simulink model "DFADAS2_SenFus_v1_201204RC_training_210115"  (R2018b)
settings: Solver=FixedStepDiscrete  StartTime=0.0  StopTime=inf  FixedStep=0.002  RelTol=1e-3  EnableMultiTasking=on
PreLoadFcn:
  | RTWConfigurationCB('preloadfcn', bdroot);
libraries: canmsglib x108, simulink x48, canfdmsglib x12
(part 20 of 28)

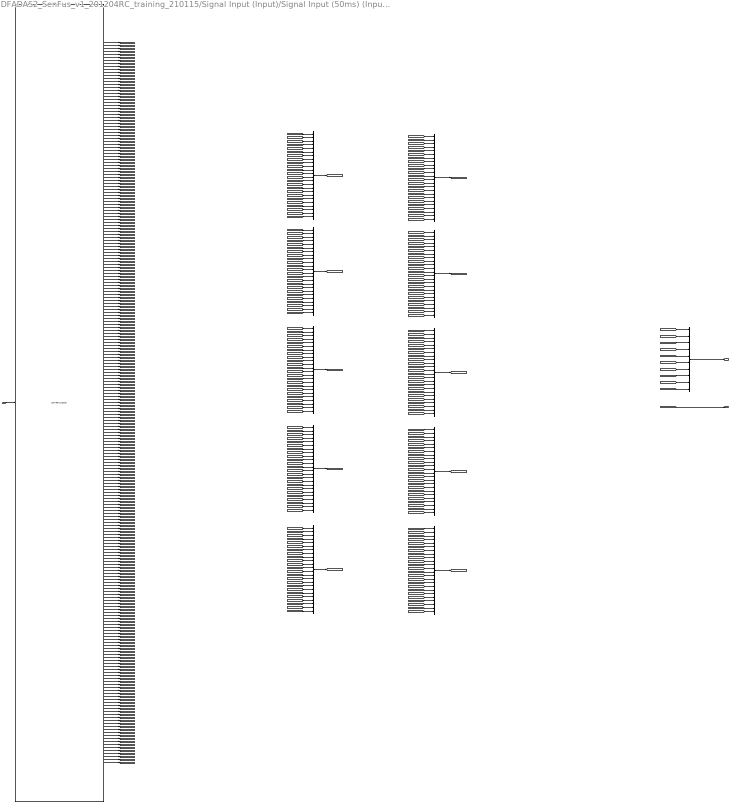
== system DFADAS2_SenFus_v1_201204RC_training_210115/Signal Input (Input)/Signal Input (50ms) (Input50)/Front Left Radar(S2) Objects Information (FLRdr)/S0 Data Frame Read/Enabled Subsystem/Unpack/If Action Subsystem/Unpack ==
  msg : Inport
  Bus Creator : BusCreator  Inputs=10
  Bus Creator{1..10} (10 alike) : BusCreator  Inputs=24
  CAN FD Unpack3 : canfdmsglib/CAN FD Unpack  CANdbFile=C:\Users\ThinkPad\Desktop\200529-海拉角雷达DBC\PR53671_DFPV_D53_HWA_SDE_F-SRR_CANFD_DF RESEARCH.dbc  MsgList=Object_Data_S2  MsgName=Object_Data_S2  ProtocolMode=CAN FD  MsgIDType=Standard (11-bit identifier)  MsgIdentifier=855  MsgLength=64  SignalInfo=ClassHighestProb_S2_001$135$7$1$2$3$0$1.000000e-02$0$-Inf$Inf$#ClassHighestProb_S2_002$323$7$1$2$3$0$1.000000e-02$0$-Inf$Inf$#ClassHighestProb_S2_003$135$7$1$2$3$1$1.000000e-02$0$-Inf$Inf$#ClassHighestProb_S2_004$323$7$1$2$3$1$1.000000e-02$0$-Inf$Inf$#ClassHighestProb_S2_005$135$7$1$2$3$2$1.000000e-02$0$-Inf$Inf$#ClassHighestProb_S2_006$323$7$1$2$3$2$1.000000e-02$0$-Inf$Inf$#ClassHighestProb_S2_007$135$7$1$2$3$3$1.000000e-02$0$-Inf$Inf$#ClassHighestProb_S2_008$323$7$1$2$3$3$1.000000e-02$0$-Inf$Inf$#ClassHighestProb_S2_009$135$7$1$2$3$4$1.000000e-02$0$-Inf$Inf$#ClassHighestProb_S2_010$323$7$1$2$3$4$1.000000e-02$0$-Inf$Inf$#ClassHighest_S2_001$132$3$1$2$3$0$1$0$0$7$#ClassHighest_S2_002$320$3$1$2$3$0$1$0$0$7$#ClassHighest_S2_003$132$3$1$2$3$1$1$0$0$7$#ClassHighest_S2_004$320$3$1$2$3$1$1$0$0$7$#ClassHighest_S2_005$132$3$1$2$3$2$1$0$0$7$#ClassHighest_S2_006$320$3$1$2$3$2$1$0$0$7$#ClassHighest_S2_007$132$3$1$2$3$3$1$0$0$7$#ClassHighest_S2_008$320$3$1$2$3$3$1$0$0$7$#ClassHighest_S2_009$132$3$1$2$3$4$1$0$0$7$#ClassHighest_S2_010$320$3$1$2$3$4$1$0$0$7$#ExistenceProbability_S2_001$121$7$1$2$3$0$1.000000e-02$0$0$1$#ExistenceProbability_S2_002$309$7$1$2$3$0$1.000000e-02$0$0$1$#ExistenceProbability_S2_003$121$7$1$2$3$1$1.000000e-02$0$0$1$#ExistenceProbability_S2_004$309$7$1$2$3$1$1.000000e-02$0$0$1$#ExistenceProbability_S2_005$121$7$1$2$3$2$1.000000e-02$0$0$1$#ExistenceProbability_S2_006$309$7$1$2$3$2$1.000000e-02$0$0$1$#ExistenceProbability_S2_007$121$7$1$2$3$3$1.000000e-02$0$0$1$#ExistenceProbability_S2_008$309$7$1$2$3$3$1.000000e-02$0$0$1$#ExistenceProbability_S2_009$121$7$1$2$3$4$1.000000e-02$0$0$1$#ExistenceProbability_S2_010$309$7$1$2$3$4$1.000000e-02$0$0$1$#Height_S2_001$146$6$1$2$3$0$1.000000e-01$0$0$5$#Height_S2_002$334$6$1$2$3$0$1.000000e-01$0$0$5$#Height_S2_003$146$6$1$2$3$1$1.000000e-01$0$0$5$#Height_S2_004$334$6$1$2$3$1$1.000000e-01$0$0$5$#Height_S2_005$146$6$1$2$3$2$1.000000e-01$0$0$5$#Height_S2_006$334$6$1$2$3$2$1.000000e-01$0$0$5$#Height_S2_007$146$6$1$2$3$3$1.000000e-01$0$0$5$#Height_S2_008$334$6$1$2$3$3$1.000000e-01$0$0$5$#Height_S2_009$146$6$1$2$3$4$1.000000e-01$0$0$5$#Height_S2_010$334$6$1$2$3$4$1.000000e-01$0$0$5$#Id_S2_001$8$10$1$2$3$0$1$1$1$1023$#Id_S2_002$196$10$1$2$3$0$1$1$1$1023$#Id_S2_003$8$10$1$2$3$1$1$1$1$1023$#Id_S2_004$196$10$1$2$3$1$1$1$1$1023$#Id_S2_005$8$10$1$2$3$2$1$1$1$1023$#Id_S2_006$196$10$1$2$3$2$1$1$1$1023$#Id_S2_007$8$10$1$2$3$3$1$1$1$1023$#Id_S2_008$196$10$1$2$3$3$1$1$1$1023$#Id_S2_009$8$10$1$2$3$4$1$1$1$1023$#Id_S2_010$196$10$1$2$3$4$1$1$1$1023$#Length_S2_001$102$9$1$2$3$0$1.000000e-01$0$3.000000e-01$5.140000e+01$#Length_S2_002$290$9$1$2$3$0$1.000000e-01$0$3.000000e-01$5.140000e+01$#Length_S2_003$102$9$1$2$3$1$1.000000e-01$0$3.000000e-01$5.140000e+01$#Length_S2_004$290$9$1$2$3$1$1.000000e-01$0$3.000000e-01$5.140000e+01$#Length_S2_005$102$9$1$2$3$2$1.000000e-01$0$3.000000e-01$5.140000e+01$#Length_S2_006$290$9$1$2$3$2$1.000000e-01$0$3.000000e-01$5.140000e+01$#Length_S2_007$102$9$1$2$3$3$1.000000e-01$0$3.000000e-01$5.140000e+01$#Length_S2_008$290$9$1$2$3$3$1.000000e-01$0$3.000000e-01$5.140000e+01$#Length_S2_009$102$9$1$2$3$4$1.000000e-01$0$3.000000e-01$5.140000e+01$#Length_S2_010$290$9$1$2$3$4$1.000000e-01$0$3.000000e-01$5.140000e+01$#MovingState_S2_001$128$4$1$2$3$0$1$0$0$15$#MovingState_S2_002$316$4$1$2$3$0$1$0$0$15$#MovingState_S2_003$128$4$1$2$3$1$1$0$0$15$#MovingState_S2_004$316$4$1$2$3$1$1$0$0$15$#MovingState_S2_005$128$4$1$2$3$2$1$0$0$15$#MovingState_S2_006$316$4$1$2$3$2$1$0$0$15$#MovingState_S2_007$128$4$1$2$3$3$1$0$0$15$#MovingState_S2_008$316$4$1$2$3$3$1$0$0$15$#MovingState_S2_009$128$4$1$2$3$4$1$0$0$15$#MovingState_S2_010$316$4$1$2$3$4$1$0$0$15$#Multiplexor$0$8$1$2$2$0$1$0$0$255$#ObjInit_S2_001$18$1$1$2$3$0$1$0$0$1$#ObjInit_S2_002$206$1$1$2$3$0$1$0$0$1$#ObjInit_S2_003$18$1$1$2$3$1$1$0$0$1$#ObjInit_S2_004$206$1$1$2$3$1$1$0$0$1$#ObjInit_S2_005$18$1$1$2$3$2$1$0$0$1$#ObjInit_S2_006$206$1$1$2$3$2$1$0$0$1$#ObjInit_S2_007$18$1$1$2$3$3$1$0$0$1$#ObjInit_S2_008$206$1$1$2$3$3$1$0$0$1$#ObjInit_S2_009$18$1$1$2$3$4$1$0$0$1$#ObjInit_S2_010$206$1$1$2$3$4$1$0$0$1$#ObjMeasured_S2_001$19$1$1$2$3$0$1$0$0$1$#ObjMeasured_S2_002$207$1$1$2$3$0$1$0$0$1$#ObjMeasured_S2_003$19$1$1$2$3$1$1$0$0$1$#ObjMeasured_S2_004$207$1$1$2$3$1$1$0$0$1$#ObjMeasured_S2_005$19$1$1$2$3$2$1$0$0$1$#ObjMeasured_S2_006$207$1$1$2$3$2$1$0$0$1$#ObjMeasured_S2_007$19$1$1$2$3$3$1$0$0$1$#ObjMeasured_S2_008$207$1$1$2$3$3$1$0$0$1$#ObjMeasured_S2_009$19$1$1$2$3$4$1$0$0$1$#ObjMeasured_S2_010$207$1$1$2$3$4$1$0$0$1$#Orientation_S2_001$111$10$1$2$3$0$1.000000e-02$-3.140000e+00$-3.140000e+00$3.140000e+00$#Orientation_S2_002$299$10$1$2$3$0$1.000000e-02$-3.140000e+00$-3.140000e+00$3.140000e+00$#Orientation_S2_003$111$10$1$2$3$1$1.000000e-02$-3.140000e+00$-3.140000e+00$3.140000e+00$#Orientation_S2_004$299$10$1$2$3$1$1.000000e-02$-3.140000e+00$-3.140000e+00$3.140000e+00$#Orientation_S2_005$111$10$1$2$3$2$1.000000e-02$-3.140000e+00$-3.140000e+00$3.140000e+00$#Orientation_S2_006$299$10$1$2$3$2$1.000000e-02$-3.140000e+00$-3.140000e+00$3.140000e+00$#Orientation_S2_007$111$10$1$2$3$3$1.000000e-02$-3.140000e+00$-3.140000e+00$3.140000e+00$#Orientation_S2_008$299$10$1$2$3$3$1.000000e-02$-3.140000e+00$-3.140000e+00$3.140000e+00$#Orientation_S2_009$111$10$1$2$3$4$1.000000e-02$-3.140000e+00$-3.140000e+00$3.140000e+00$#Orientation_S2_010$299$10$1$2$3$4$1.000000e-02$-3.140000e+00$-3.140000e+00$3.140000e+00$#ReferencePoint_S2_001$142$4$1$2$3$0$1$0$0$9$#ReferencePoint_S2_002$330$4$1$2$3$0$1$0$0$9$#ReferencePoint_S2_003$142$4$1$2$3$1$1$0$0$9$#ReferencePoint_S2_004$330$4$1$2$3$1$1$0$0$9$#ReferencePoint_S2_005$142$4$1$2$3$2$1$0$0$9$#ReferencePoint_S2_006$330$4$1$2$3$2$1$0$0$9$#ReferencePoint_S2_007$142$4$1$2$3$3$1$0$0$9$#ReferencePoint_S2_008$330$4$1$2$3$3$1$0$0$9$#ReferencePoint_S2_009$142$4$1$2$3$4$1$0$0$9$#ReferencePoint_S2_010$330$4$1$2$3$4$1$0$0$9$#Width_S2_001$97$5$1$2$3$0$1.000000e-01$0$3.000000e-01$3.300000e+00$#Width_S2_002$285$5$1$2$3$0$1.000000e-01$0$3.000000e-01$3.300000e+00$#Width_S2_003$97$5$1$2$3$1$1.000000e-01$0$3.000000e-01$3.300000e+00$#Width_S2_004$285$5$1$2$3$1$1.000000e-01$0$3.000000e-01$3.300000e+00$#Width_S2_005$97$5$1$2$3$2$1.000000e-01$0$3.000000e-01$3.300000e+00$#Width_S2_006$285$5$1$2$3$2$1.000000e-01$0$3.000000e-01$3.300000e+00$#Width_S2_007$97$5$1$2$3$3$1.000000e-01$0$3.000000e-01$3.300000e+00$#Width_S2_008$285$5$1$2$3$3$1.000000e-01$0$3.000000e-01$3.300000e+00$#Width_S2_009$97$5$1$2$3$4$1.000000e-01$0$3.000000e-01$3.300000e+00$#Width_S2_010$285$5$1$2$3$4$1.000000e-01$0$3.000000e-01$3.300000e+00$#XAccelerationStd_S2_001$152$6$1$2$3$0$1$0$0$5$#XAccelerationStd_S2_002$340$6$1$2$3$0$1$0$0$5$#XAccelerationStd_S2_003$152$6$1$2$3$1$1$0$0$5$#XAccelerationStd_S2_004$340$6$1$2$3$1$1$0$0$5$#XAccelerationStd_S2_005$152$6$1$2$3$2$1$0$0$5$#XAccelerationStd_S2_006$340$6$1$2$3$2$1$0$0$5$#XAccelerationStd_S2_007$152$6$1$2$3$3$1$0$0$5$#XAccelerationStd_S2_008$340$6$1$2$3$3$1$0$0$5$#XAccelerationStd_S2_009$152$6$1$2$3$4$1$0$0$5$#XAccelerationStd_S2_010$340$6$1$2$3$4$1$0$0$5$#XAcceleration_S2_001$79$9$1$2$3$0$1.000000e-01$-2.560000e+01$-2.560000e+01$2.550000e+01$#XAcceleration_S2_002$267$9$1$2$3$0$1.000000e-01$-2.560000e+01$-2.560000e+01$2.550000e+01$#XAcceleration_S2_003$79$9$1$2$3$1$1.000000e-01$-2.560000e+01$-2.560000e+01$2.550000e+01$#XAcceleration_S2_004$267$9$1$2$3$1$1.000000e-01$-2.560000e+01$-2.560000e+01$2.550000e+01$#XAcceleration_S2_005$79$9$1$2$3$2$1.000000e-01$-2.560000e+01$-2.560000e+01$2.550000e+01$#XAcceleration_S2_006$267$9$1$2$3$2$1.000000e-01$-2.560000e+01$-2.560000e+01$2.550000e+01$#XAcceleration_S2_007$79$9$1$2$3$3$1.000000e-01$-2.560000e+01$-2.560000e+01$2.550000e+01$#XAcceleration_S2_008$267$9$1$2$3$3$1.000000e-01$-2.560000e+01$-2.560000e+01$2.550000e+01$#XAcceleration_S2_009$79$9$1$2$3$4$1.000000e-01$-2.560000e+01$-2.560000e+01$2.550000e+01$#XAcceleration_S2_010$267$9$1$2$3$4$1.000000e-01$-2.560000e+01$-2.560000e+01$2.550000e+01$#XPosStd_S2_001$158$8$1$2$3$0$1.000000e-01$0$0$25$#XPosStd_S2_002$346$8$1$2$3$0$1.000000e-01$0$0$25$#XPosStd_S2_003$158$8$1$2$3$1$1.000000e-01$0$0$25$#XPosStd_S2_004$346$8$1$2$3$1$1.000000e-01$0$0$25$#XPosStd_S2_005$158$8$1$2$3$2$1.000000e-01$0$0$25$#XPosStd_S2_006$346$8$1$2$3$2$1.000000e-01$0$0$25$#XPosStd_S2_007$158$8$1$2$3$3$1.000000e-01$0$0$25$#XPosStd_S2_008$346$8$1$2$3$3$1.000000e-01$0$0$25$#XPosStd_S2_009$158$8$1$2$3$4$1.000000e-01$0$0$25$#XPosStd_S2_010$346$8$1$2$3$4$1.000000e-01$0$0$25$#XPos_S2_001$20$16$1$2$3$0$1.000000e-02$-3.276800e+02$-3.276800e+02$3.276700e+02$#XPos_S2_002$208$16$1$2$3$0$1.000000e-02$-3.276800e+02$-3.276800e+02$3.276700e+02$#XPos_S2_003$20$16$1$2$3$1$1.000000e-02$-3.276800e+02$-3.276800e+02$3.276700e+02$#XPos_S2_004$208$16$1$2$3$1$1.000000e-02$-3.276800e+02$-3.276800e+02$3.276700e+02$#XPos_S2_005$20$16$1$2$3$2$1.000000e-02$-3.276800e+02$-3.276800e+02$3.276700e+02$#XPos_S2_006$208$16$1$2$3$2$1.000000e-02$-3.276800e+02$-3.276800e+02$3.276700e+02$#XPos_S2_007$20$16$1$2$3$3$1.000000e-02$-3.276800e+02$-3.276800e+02$3.276700e+02$#XPos_S2_008$208$16$1$2$3$3$1.000000e-02$-3.276800e+02$-3.276800e+02$3.276700e+02$#XPos_S2_009$20$16$1$2$3$4$1.000000e-02$-3.276800e+02$-3.276800e+02$3.276700e+02$#XPos_S2_010$208$16$1$2$3$4$1.000000e-02$-3.276800e+02$-3.276800e+02$3.276700e+02$#XVelocityStd_S2_001$166$8$1$2$3$0$1.000000e-01$0$0$15$#XVelocityStd_S2_002$354$8$1$2$3$0$1.000000e-01$0$0$15$#XVelocityStd_S2_003$166$8$1$2$3$1$1.000000e-01$0$0$15$#XVelocityStd_S2_004$354$8$1$2$3$1$1.000000e-01$0$0$15$#XVelocityStd_S2_005$166$8$1$2$3$2$1.000000e-01$0$0$15$#XVelocityStd_S2_006$354$8$1$2$3$2$1.000000e-01$0$0$15$#XVelocityStd_S2_007$166$8$1$2$3$3$1.000000e-01$0$0$15$#XVelocityStd_S2_008$354$8$1$2$3$3$1.000000e-01$0$0$15$#XVelocityStd_S2_009$166$8$1$2$3$4$1.000000e-01$0$0$15$#XVelocityStd_S2_010$354$8$1$2$3$4$1.000000e-01$0$0$15$#XVelocity_S2_001$51$14$1$2$3$0$1.000000e-02$-8.192000e+01$-8.192000e+01$8.191000e+01$#XVelocity_S2_002$239$14$1$2$3$0$1.000000e-02$-8.192000e+01$-8.192000e+01$8.191000e+01$#XVelocity_S2_003$51$14$1$2$3$1$1.000000e-02$-8.192000e+01$-8.192000e+01$8.191000e+01$#XVelocity_S2_004$239$14$1$2$3$1$1.000000e-02$-8.192000e+01$-8.192000e+01$8.191000e+01$#XVelocity_S2_005$51$14$1$2$3$2$1.000000e-02$-8.192000e+01$-8.192000e+01$8.191000e+01$#XVelocity_S2_006$239$14$1$2$3$2$1.000000e-02$-8.192000e+01$-8.192000e+01$8.191000e+01$#XVelocity_S2_007$51$14$1$2$3$3$1.000000e-02$-8.192000e+01$-8.192000e+01$8.191000e+01$#XVelocity_S2_008$239$14$1$2$3$3$1.000000e-02$-8.192000e+01$-8.192000e+01$8.191000e+01$#XVelocity_S2_009$51$14$1$2$3$4$1.000000e-02$-8.192000e+01$-8.192000e+01$8.191000e+01$#XVelocity_S2_010$239$14$1$2$3$4$1.000000e-02$-8.192000e+01$-8.192000e+01$8.191000e+01$#YAccelerationStd_S2_001$174$6$1$2$3$0$1.000000e-01$0$0$5$#YAccelerationStd_S2_002$362$6$1$2$3$0$1.000000e-01$0$0$5$#YAccelerationStd_S2_003$174$6$1$2$3$1$1.000000e-01$0$0$5$#YAccelerationStd_S2_004$362$6$1$2$3$1$1.000000e-01$0$0$5$#YAccelerationStd_S2_005$174$6$1$2$3$2$1.000000e-01$0$0$5$#YAccelerationStd_S2_006$362$6$1$2$3$2$1.000000e-01$0$0$5$#YAccelerationStd_S2_007$174$6$1$2$3$3$1.000000e-01$0$0$5$#YAccelerationStd_S2_008$362$6$1$2$3$3$1.000000e-01$0$0$5$#YAccelerationStd_S2_009$174$6$1$2$3$4$1.000000e-01$0$0$5$#YAccelerationStd_S2_010$362$6$1$2$3$4$1.000000e-01$0$0$5$#YAcceleration_S2_001$88$9$1$2$3$0$1.000000e-01$-2.560000e+01$-2.560000e+01$2.550000e+01$#YAcceleration_S2_002$276$9$1$2$3$0$1.000000e-01$-2.560000e+01$-2.560000e+01$2.550000e+01$#YAcceleration_S2_003$88$9$1$2$3$1$1.000000e-01$-2.560000e+01$-2.560000e+01$2.550000e+01$#YAcceleration_S2_004$276$9$1$2$3$1$1.000000e-01$-2.560000e+01$-2.560000e+01$2.550000e+01$#YAcceleration_S2_005$88$9$1$2$3$2$1.000000e-01$-2.560000e+01$-2.560000e+01$2.550000e+01$#YAcceleration_S2_006$276$9$1$2$3$2$1.000000e-01$-2.560000e+01$-2.560000e+01$2.550000e+01$#YAcceleration_S2_007$88$9$1$2$3$3$1.000000e-01$-2.560000e+01$-2.560000e+01$2.550000e+01$#YAcceleration_S2_008$276$9$1$2$3$3$1.000000e-01$-2.560000e+01$-2.560000e+01$2.550000e+01$#YAcceleration_S2_009$88$9$1$2$3$4$1.000000e-01$-2.560000e+01$-2.560000e+01$2.550000e+01$#YAcceleration_S2_010$276$9$1$2$3$4$1.000000e-01$-2.560000e+01$-2.560000e+01$2.550000e+01$#YPosStd_S2_001$180$8$1$2$3$0$1.000000e-01$0$0$25$#YPosStd_S2_002$368$8$1$2$3$0$1.000000e-01$0$0$25$#YPosStd_S2_003$180$8$1$2$3$1$1.000000e-01$0$0$25$#YPosStd_S2_004$368$8$1$2$3$1$1.000000e-01$0$0$25$#YPosStd_S2_005$180$8$1$2$3$2$1.000000e-01$0$0$25$#YPosStd_S2_006$368$8$1$2$3$2$1.000000e-01$0$0$25$#YPosStd_S2_007$180$8$1$2$3$3$1.000000e-01$0$0$25$#YPosStd_S2_008$368$8$1$2$3$3$1.000000e-01$0$0$25$#YPosStd_S2_009$180$8$1$2$3$4$1.000000e-01$0$0$25$#YPosStd_S2_010$368$8$1$2$3$4$1.000000e-01$0$0$25$#YPos_S2_001$36$15$1$2$3$0$1.000000e-02$-1.638400e+02$-1.638400e+02$1.638300e+02$#YPos_S2_002$224$15$1$2$3$0$1.000000e-02$-1.638400e+02$-1.638400e+02$1.638300e+02$#YPos_S2_003$36$15$1$2$3$1$1.000000e-02$-1.638400e+02$-1.638400e+02$1.638300e+02$#YPos_S2_004$224$15$1$2$3$1$1.000000e-02$-1.638400e+02$-1.638400e+02$1.638300e+02$#YPos_S2_005$36$15$1$2$3$2$1.000000e-02$-1.638400e+02$-1.638400e+02$1.638300e+02$#YPos_S2_006$224$15$1$2$3$2$1.000000e-02$-1.638400e+02$-1.638400e+02$1.638300e+02$#YPos_S2_007$36$15$1$2$3$3$1.000000e-02$-1.638400e+02$-1.638400e+02$1.638300e+02$#YPos_S2_008$224$15$1$2$3$3$1.000000e-02$-1.638400e+02$-1.638400e+02$1.638300e+02$#YPos_S2_009$36$15$1$2$3$4$1.000000e-02$-1.638400e+02$-1.638400e+02$1.638300e+02$#YPos_S2_010$224$15$1$2$3$4$1.000000e-02$-1.638400e+02$-1.638400e+02$1.638300e+02$#YVelocityStd_S2_001$188$8$1$2$3$0$1.000000e-01$0$0$15$#YVelocityStd_S2_002$376$8$1$2$3$0$1.000000e-01$0$0$15$#YVelocityStd_S2_003$188$8$1$2$3$1$1.000000e-01$0$0$15$#YVelocityStd_S2_004$376$8$1$2$3$1$1.000000e-01$0$0$15$#YVelocityStd_S2_005$188$8$1$2$3$2$1.000000e-01$0$0$15$#YVelocityStd_S2_006$376$8$1$2$3$2$1.000000e-01$0$0$15$#YVelocityStd_S2_007$188$8$1$2$3$3$1.000000e-01$0$0$15$#YVelocityStd_S2_008$376$8$1$2$3$3$1.000000e-01$0$0$15$#YVelocityStd_S2_009$188$8$1$2$3$4$1.000000e-01$0$0$15$#YVelocityStd_S2_010$376$8$1$2$3$4$1.000000e-01$0$0$15$#YVelocity_S2_001$65$14$1$2$3$0$1.000000e-02$-8.192000e+01$-8.192000e+01$8.191000e+01$#YVelocity_S2_002$253$14$1$2$3$0$1.000000e-02$-8.192000e+01$-8.192000e+01$8.191000e+01$#YVelocity_S2_003$65$14$1$2$3$1$1.000000e-02$-8.192000e+01$-8.192000e+01$8.191000e+01$#YVelocity_S2_004$253$14$1$2$3$1$1.000000e-02$-8.192000e+01$-8.192000e+01$8.191000e+01$#YVelocity_S2_005$65$14$1$2$3$2$1.000000e-02$-8.192000e+01$-8.192000e+01$8.191000e+01$#YVelocity_S2_006$253$14$1$2$3$2$1.000000e-02$-8.192000e+01$-8.192000e+01$8.191000e+01$#YVelocity_S2_007$65$14$1$2$3$3$1.000000e-02$-8.192000e+01$-8.192000e+01$8.191000e+01$#YVelocity_S2_008$253$14$1$2$3$3$1.000000e-02$-8.192000e+01$-8.192000e+01$8.191000e+01$#YVelocity_S2_009$65$14$1$2$3$4$1.000000e-02$-8.192000e+01$-8.192000e+01$8.191000e+01$#YVelocity_S2_010$253$14$1$2$3$4$1.000000e-02$-8.192000e+01$-8.192000e+01$8.191000e+01$#  NSignals=241  IDPort=off  TimestampPort=off  ErrorPort=off  RemotePort=off  LengthPort=off  StatusPort=off  BRSPort=off  ESIPort=off  DLCPort=off  StartBits=str2num('[int32(135);int32(323);int32(135);int32(323);int32(135);int32(323);int32(135);int32(323);int32(135);int32(323);int32(132);int32(320);int32(132);int32(320);int32(132);int32(320);int32(132);int32(320);int32(132);int32(320);int32(121);int32(309);int32(121);int32(309);int32(121);int32(309);int32(121);int32(309);int32(121);int32(309);int32(146);int32(334);int32(146);int32(334);int32(146);int32(334);int32(146);int32(334);int32(146);int32(334);int32(8);int32(196);int32(8);int32(196);int32(8);int32(196);int32(8);int32(196);int32(8);int32(196);int32(102);int32(290);int32(102);int32(290);int32(102);int32(290);int32(102);int32(290);int32(102);int32(290);int32(128);int32(316);int32(128);int32(316);int32(128);int32(316);int32(128);int32(316);int32(128);int32(316);int32(0);int32(18);int32(206);int32(18);int32(206);int32(18);int32(206);int32(18);int32(206);int32(18);int32(206);int32(19);int32(207);int32(19);int32(207);int32(19);int32(207);int32(19);int32(207);int32(19);int32(207);int32(111);int32(299);int32(111);int32(299);int32(111);int32(299);int32(111);int32(299);int32(111);int32(299);int32(142);int32(330);int32(142);int32(330);int32(142);int32(330);int32(142);int32(330);int32(142);int32(330);int32(97);int32(285);int32(97);int32(285);int32(97);int32(285);int32(97);int32(285);int32(97);int32(285);int32(152);int32(340);int32(152);int32(340);int32(152);int32(340);int32(152);int32(340);int32(152);int32(340);int32(79);int32(267);int32(79);int32(267);int32(79);int32(267);int32(79);int32(267);int32(79);int32(267);int32(158);int32(346);int32(158);int32(346);int32(158);int32(346);int32(158);int32(346);int32(158);int32(346);int32(20);int32(208);int32(20);int32(208);int32(20);int32(208);int32(20);int32(208);int32(20);int32(208);int32(166);int32(354);int32(166);int32(354);int32(166);int32(354);int32(166);int32(354);int32(166);int32(354);int32(51);int32(239);int32(51);int32(239);int32(51);int32(239);int32(51);int32(239);int32(51);int32(239);int32(174);int32(362);int32(174);int32(362);int32(174);int32(362);int32(174);int32(362);int32(174);int32(362);int32(88);int32(276);int32(88);int32(276);int32(88);int32(276);int32(88);int32(276);int32(88);int32(276);int32(180);int32(368);int32(180);int32(368);int32(180);int32(368);int32(180);int32(368);int32(180);int32(368);int32(36);int32(224);int32(36);int32(224);int32(36);int32(224);int32(36);int32(224);int32(36);int32(224);int32(188);int32(376);int32(188);int32(376);int32(188);int32(376);int32(188);int32(376);int32(188);int32(376);int32(65);int32(253);int32(65);int32(253);int32(65);int32(253);int32(65);int32(253);int32(65);int32(253)]')  SignalSizes=str2num('[int32(7);int32(7);int32(7);int32(7);int32(7);int32(7);int32(7);int32(7);int32(7);int32(7);int32(3);int32(3);int32(3);int32(3);int32(3);int32(3);int32(3);int32(3);int32(3);int32(3);int32(7);int32(7);int32(7);int32(7);int32(7);int32(7);int32(7);int32(7);int32(7);int32(7);int32(6);int32(6);int32(6);int32(6);int32(6);int32(6);int32(6);int32(6);int32(6);int32(6);int32(10);int32(10);int32(10);int32(10);int32(10);int32(10);int32(10);int32(10);int32(10);int32(10);int32(9);int32(9);int32(9);int32(9);int32(9);int32(9);int32(9);int32(9);int32(9);int32(9);int32(4);int32(4);int32(4);int32(4);int32(4);int32(4);int32(4);int32(4);int32(4);int32(4);int32(8);int32(1);int32(1);int32(1);int32(1);int32(1);int32(1);int32(1);int32(1);int32(1);int32(1);int32(1);int32(1);int32(1);int32(1);int32(1);int32(1);int32(1);int32(1);int32(1);int32(1);int32(10);int32(10);int32(10);int32(10);int32(10);int32(10);int32(10);int32(10);int32(10);int32(10);int32(4);int32(4);int32(4);int32(4);int32(4);int32(4);int32(4);int32(4);int32(4);int32(4);int32(5);int32(5);int32(5);int32(5);int32(5);int32(5);int32(5);int32(5);int32(5);int32(5);int32(6);int32(6);int32(6);int32(6);int32(6);int32(6);int32(6);int32(6);int32(6);int32(6);int32(9);int32(9);int32(9);int32(9);int32(9);int32(9);int32(9);int32(9);int32(9);int32(9);int32(8);int32(8);int32(8);int32(8);int32(8);int32(8);int32(8);int32(8);int32(8);int32(8);int32(16);int32(16);int32(16);int32(16);int32(16);int32(16);int32(16);int32(16);int32(16);int32(16);int32(8);int32(8);int32(8);int32(8);int32(8);int32(8);int32(8);int32(8);int32(8);int32(8);int32(14);int32(14);int32(14);int32(14);int32(14);int32(14);int32(14);int32(14);int32(14);int32(14);int32(6);int32(6);int32(6);int32(6);int32(6);int32(6);int32(6);int32(6);int32(6);int32(6);int32(9);int32(9);int32(9);int32(9);int32(9);int32(9);int32(9);int32(9);int32(9);int32(9);int32(8);int32(8);int32(8);int32(8);int32(8);int32(8);int32(8);int32(8);int32(8);int32(8);int32(15);int32(15);int32(15);int32(15);int32(15);int32(15);int32(15);int32(15);int32(15);int32(15);int32(8);int32(8);int32(8);int32(8);int32(8);int32(8);int32(8);int32(8);int32(8);int32(8);int32(14);int32(14);int32(14);int32(14);int32(14);int32(14);int32(14);int32(14);int32(14);int32(14)]')  ByteOrders=str2num('[int32(1);int32(1);int32(1);int32(1);int32(1);int32(1);int32(1);int32(1);int32(1);int32(1);int32(1);int32(1);int32(1);int32(1);int32(1);int32(1);int32(1);int32(1);int32(1);int32(1);int32(1);int32(1);int32(1);int32(1);int32(1);int32(1);int32(1);int32(1);int32(1);int32(1);int32(1);int32(1);int32(1);int32(1);int32(1);int32(1);int32(1);int32(1);int32(1);int32(1);int32(1);int32(1);int32(1);int32(1);int32(1);int32(1);int32(1);int32(1);int32(1);int32(1);int32(1);int32(1);int32(1);int32(1);int32(1);int32(1);int32(1);int32(1);int32(1);int32(1);int32(1);int32(1);int32(1);int32(1);int32(1);int32(1);int32(1);int32(1);int32(1);int32(1);int32(1);int32(1);int32(1);int32(1);int32(1);int32(1);int32(1);int32(1);int32(1);int32(1);int32(1);int32(1);int32(1);int32(1);int32(1);int32(1);int32(1);int32(1);int32(1);int32(1);int32(1);int32(1);int32(1);int32(1);int32(1);int32(1);int32(1);int32(1);int32(1);int32(1);int32(1);int32(1);int32(1);int32(1);int32(1);int32(1);int32(1);int32(1);int32(1);int32(1);int32(1);int32(1);int32(1);int32(1);int32(1);int32(1);int32(1);int32(1);int32(1);int32(1);int32(1);int32(1);int32(1);int32(1);int32(1);int32(1);int32(1);int32(1);int32(1);int32(1);int32(1);int32(1);int32(1);int32(1);int32(1);int32(1);int32(1);int32(1);int32(1);int32(1);int32(1);int32(1);int32(1);int32(1);int32(1);int32(1);int32(1);int32(1);int32(1);int32(1);int32(1);int32(1);int32(1);int32(1);int32(1);int32(1);int32(1);int32(1);int32(1);int32(1);int32(1);int32(1);int32(1);int32(1);int32(1);int32(1);int32(1);int32(1);int32(1);int32(1);int32(1);int32(1);int32(1);int32(1);int32(1);int32(1);int32(1);int32(1);int32(1);int32(1);int32(1);int32(1);int32(1);int32(1);int32(1);int32(1);int32(1);int32(1);int32(1);int32(1);int32(1);int32(1);int32(1);int32(1);int32(1);int32(1);int32(1);int32(1);int32(1);int32(1);int32(1);int32(1);int32(1);int32(1);int32(1);int32(1);int32(1);int32(1);int32(1);int32(1);int32(1);int32(1);int32(1);int32(1);int32(1);int32(1);int32(1);int32(1);int32(1);int32(1);int32(1);int32(1);int32(1);int32(1);int32(1);int32(1);int32(1);int32(1);int32(1);int32(1);int32(1);int32(1);int32(1);int32(1);int32(1);int32(1);int32(1);int32(1);int32(1);int32(1);int32(1)]')  DataTypes=str2num('[int32(2);int32(2);int32(2);int32(2);int32(2);int32(2);int32(2);int32(2);int32(2);int32(2);int32(2);int32(2);int32(2);int32(2);int32(2);int32(2);int32(2);int32(2);int32(2);int32(2);int32(2);int32(2);int32(2);int32(2);int32(2);int32(2);int32(2);int32(2);int32(2);int32(2);int32(2);int32(2);int32(2);int32(2);int32(2);int32(2);int32(2);int32(2);int32(2);int32(2);int32(2);int32(2);int32(2);int32(2);int32(2);int32(2);int32(2);int32(2);int32(2);int32(2);int32(2);int32(2);int32(2);int32(2);int32(2);int32(2);int32(2);int32(2);int32(2);int32(2);int32(2);int32(2);int32(2);int32(2);int32(2);int32(2);int32(2);int32(2);int32(2);int32(2);int32(2);int32(2);int32(2);int32(2);int32(2);int32(2);int32(2);int32(2);int32(2);int32(2);int32(2);int32(2);int32(2);int32(2);int32(2);int32(2);int32(2);int32(2);int32(2);int32(2);int32(2);int32(2);int32(2);int32(2);int32(2);int32(2);int32(2);int32(2);int32(2);int32(2);int32(2);int32(2);int32(2);int32(2);int32(2);int32(2);int32(2);int32(2);int32(2);int32(2);int32(2);int32(2);int32(2);int32(2);int32(2);int32(2);int32(2);int32(2);int32(2);int32(2);int32(2);int32(2);int32(2);int32(2);int32(2);int32(2);int32(2);int32(2);int32(2);int32(2);int32(2);int32(2);int32(2);int32(2);int32(2);int32(2);int32(2);int32(2);int32(2);int32(2);int32(2);int32(2);int32(2);int32(2);int32(2);int32(2);int32(2);int32(2);int32(2);int32(2);int32(2);int32(2);int32(2);int32(2);int32(2);int32(2);int32(2);int32(2);int32(2);int32(2);int32(2);int32(2);int32(2);int32(2);int32(2);int32(2);int32(2);int32(2);int32(2);int32(2);int32(2);int32(2);int32(2);int32(2);int32(2);int32(2);int32(2);int32(2);int32(2);int32(2);int32(2);int32(2);int32(2);int32(2);int32(2);int32(2);int32(2);int32(2);int32(2);int32(2);int32(2);int32(2);int32(2);int32(2);int32(2);int32(2);int32(2);int32(2);int32(2);int32(2);int32(2);int32(2);int32(2);int32(2);int32(2);int32(2);int32(2);int32(2);int32(2);int32(2);int32(2);int32(2);int32(2);int32(2);int32(2);int32(2);int32(2);int32(2);int32(2);int32(2);int32(2);int32(2);int32(2);int32(2);int32(2);int32(2);int32(2);int32(2);int32(2);int32(2);int32(2);int32(2);int32(2);int32(2);int32(2);int32(2);int32(2);int32(2);int32(2);int32(2);int32(2)]')  MultiplexTypes=str2num('[int32(3);int32(3);int32(3);int32(3);int32(3);int32(3);int32(3);int32(3);int32(3);int32(3);int32(3);int32(3);int32(3);int32(3);int32(3);int32(3);int32(3);int32(3);int32(3);int32(3);int32(3);int32(3);int32(3);int32(3);int32(3);int32(3);int32(3);int32(3);int32(3);int32(3);int32(3);int32(3);int32(3);int32(3);int32(3);int32(3);int32(3);int32(3);int32(3);int32(3);int32(3);int32(3);int32(3);int32(3);int32(3);int32(3);int32(3);int32(3);int32(3);int32(3);int32(3);int32(3);int32(3);int32(3);int32(3);int32(3);int32(3);int32(3);int32(3);int32(3);int32(3);int32(3);int32(3);int32(3);int32(3);int32(3);int32(3);int32(3);int32(3);int32(3);int32(2);int32(3);int32(3);int32(3);int32(3);int32(3);int32(3);int32(3);int32(3);int32(3);int32(3);int32(3);int32(3);int32(3);int32(3);int32(3);int32(3);int32(3);int32(3);int32(3);int32(3);int32(3);int32(3);int32(3);int32(3);int32(3);int32(3);int32(3);int32(3);int32(3);int32(3);int32(3);int32(3);int32(3);int32(3);int32(3);int32(3);int32(3);int32(3);int32(3);int32(3);int32(3);int32(3);int32(3);int32(3);int32(3);int32(3);int32(3);int32(3);int32(3);int32(3);int32(3);int32(3);int32(3);int32(3);int32(3);int32(3);int32(3);int32(3);int32(3);int32(3);int32(3);int32(3);int32(3);int32(3);int32(3);int32(3);int32(3);int32(3);int32(3);int32(3);int32(3);int32(3);int32(3);int32(3);int32(3);int32(3);int32(3);int32(3);int32(3);int32(3);int32(3);int32(3);int32(3);int32(3);int32(3);int32(3);int32(3);int32(3);int32(3);int32(3);int32(3);int32(3);int32(3);int32(3);int32(3);int32(3);int32(3);int32(3);int32(3);int32(3);int32(3);int32(3);int32(3);int32(3);int32(3);int32(3);int32(3);int32(3);int32(3);int32(3);int32(3);int32(3);int32(3);int32(3);int32(3);int32(3);int32(3);int32(3);int32(3);int32(3);int32(3);int32(3);int32(3);int32(3);int32(3);int32(3);int32(3);int32(3);int32(3);int32(3);int32(3);int32(3);int32(3);int32(3);int32(3);int32(3);int32(3);int32(3);int32(3);int32(3);int32(3);int32(3);int32(3);int32(3);int32(3);int32(3);int32(3);int32(3);int32(3);int32(3);int32(3);int32(3);int32(3);int32(3);int32(3);int32(3);int32(3);int32(3);int32(3);int32(3);int32(3);int32(3);int32(3);int32(3);int32(3);int32(3);int32(3);int32(3);int32(3);int32(3)]')  MultiplexValues=str2num('[double(0);double(0);double(1);double(1);double(2);double(2);double(3);double(3);double(4);double(4);double(0);double(0);double(1);double(1);double(2);double(2);double(3);double(3);double(4);double(4);double(0);double(0);double(1);double(1);double(2);double(2);double(3);double(3);double(4);double(4);double(0);double(0);double(1);double(1);double(2);double(2);double(3);double(3);double(4);double(4);double(0);double(0);double(1);double(1);double(2);double(2);double(3);double(3);double(4);double(4);double(0);double(0);double(1);double(1);double(2);double(2);double(3);double(3);double(4);double(4);double(0);double(0);double(1);double(1);double(2);double(2);double(3);double(3);double(4);double(4);double(0);double(0);double(0);double(1);double(1);double(2);double(2);double(3);double(3);double(4);double(4);double(0);double(0);double(1);double(1);double(2);double(2);double(3);double(3);double(4);double(4);double(0);double(0);double(1);double(1);double(2);double(2);double(3);double(3);double(4);double(4);double(0);double(0);double(1);double(1);double(2);double(2);double(3);double(3);double(4);double(4);double(0);double(0);double(1);double(1);double(2);double(2);double(3);double(3);double(4);double(4);double(0);double(0);double(1);double(1);double(2);double(2);double(3);double(3);double(4);double(4);double(0);double(0);double(1);double(1);double(2);double(2);double(3);double(3);double(4);double(4);double(0);double(0);double(1);double(1);double(2);double(2);double(3);double(3);double(4);double(4);double(0);double(0);double(1);double(1);double(2);double(2);double(3);double(3);double(4);double(4);double(0);double(0);double(1);double(1);double(2);double(2);double(3);double(3);double(4);double(4);double(0);double(0);double(1);double(1);double(2);double(2);double(3);double(3);double(4);double(4);double(0);double(0);double(1);double(1);double(2);double(2);double(3);double(3);double(4);double(4);double(0);double(0);double(1);double(1);double(2);double(2);double(3);double(3);double(4);double(4);double(0);double(0);double(1);double(1);double(2);double(2);double(3);double(3);double(4);double(4);double(0);double(0);double(1);double(1);double(2);double(2);double(3);double(3);double(4);double(4);double(0);double(0);double(1);double(1);double(2);double(2);double(3);double(3);double(4);double(4);double(0);double(0);double(1);double(1);double(2);double(2);double(3);double(3);double(4);double(4)]')  Factors=str2num('[double(1.000000e-02);double(1.000000e-02);double(1.000000e-02);double(1.000000e-02);double(1.000000e-02);double(1.000000e-02);double(1.000000e-02);double(1.000000e-02);double(1.000000e-02);double(1.000000e-02);double(1);double(1);double(1);double(1);double(1);double(1);double(1);double(1);double(1);double(1);double(1.000000e-02);double(1.000000e-02);double(1.000000e-02);double(1.000000e-02);double(1.000000e-02);double(1.000000e-02);double(1.000000e-02);double(1.000000e-02);double(1.000000e-02);double(1.000000e-02);double(1.000000e-01);double(1.000000e-01);double(1.000000e-01);double(1.000000e-01);double(1.000000e-01);double(1.000000e-01);double(1.000000e-01);double(1.000000e-01);double(1.000000e-01);double(1.000000e-01);double(1);double(1);double(1);double(1);double(1);double(1);double(1);double(1);double(1);double(1);double(1.000000e-01);double(1.000000e-01);double(1.000000e-01);double(1.000000e-01);double(1.000000e-01);double(1.000000e-01);double(1.000000e-01);double(1.000000e-01);double(1.000000e-01);double(1.000000e-01);double(1);double(1);double(1);double(1);double(1);double(1);double(1);double(1);double(1);double(1);double(1);double(1);double(1);double(1);double(1);double(1);double(1);double(1);double(1);double(1);double(1);double(1);double(1);double(1);double(1);double(1);double(1);double(1);double(1);double(1);double(1);double(1.000000e-02);double(1.000000e-02);double(1.000000e-02);double(1.000000e-02);double(1.000000e-02);double(1.000000e-02);double(1.000000e-02);double(1.000000e-02);double(1.000000e-02);double(1.000000e-02);double(1);double(1);double(1);double(1);double(1);double(1);double(1);double(1);double(1);double(1);double(1.000000e-01);double(1.000000e-01);double(1.000000e-01);double(1.000000e-01);double(1.000000e-01);double(1.000000e-01);double(1.000000e-01);double(1.000000e-01);double(1.000000e-01);double(1.000000e-01);double(1);double(1);double(1);double(1);double(1);double(1);double(1);double(1);double(1);double(1);double(1.000000e-01);double(1.000000e-01);double(1.000000e-01);double(1.000000e-01);double(1.000000e-01);double(1.000000e-01);double(1.000000e-01);double(1.000000e-01);double(1.000000e-01);double(1.000000e-01);double(1.000000e-01);double(1.000000e-01);double(1.000000e-01);double(1.000000e-01);double(1.000000e-01);double(1.000000e-01);double(1.000000e-01);double(1.000000e-01);double(1.000000e-01);double(1.000000e-01);double(1.000000e-02);double(1.000000e-02);double(1.000000e-02);double(1.000000e-02);double(1.000000e-02);double(1.000000e-02);double(1.000000e-02);double(1.000000e-02);double(1.000000e-02);double(1.000000e-02);double(1.000000e-01);double(1.000000e-01);double(1.000000e-01);double(1.000000e-01);double(1.000000e-01);double(1.000000e-01);double(1.000000e-01);double(1.000000e-01);double(1.000000e-01);double(1.000000e-01);double(1.000000e-02);double(1.000000e-02);double(1.000000e-02);double(1.000000e-02);double(1.000000e-02);double(1.000000e-02);double(1.000000e-02);double(1.000000e-02);double(1.000000e-02);double(1.000000e-02);double(1.000000e-01);double(1.000000e-01);double(1.000000e-01);double(1.000000e-01);double(1.000000e-01);double(1.000000e-01);double(1.000000e-01);double(1.000000e-01);double(1.000000e-01);double(1.000000e-01);double(1.000000e-01);double(1.000000e-01);double(1.000000e-01);double(1.000000e-01);double(1.000000e-01);double(1.000000e-01);double(1.000000e-01);double(1.000000e-01);double(1.000000e-01);double(1.000000e-01);double(1.000000e-01);double(1.000000e-01);double(1.000000e-01);double(1.000000e-01);double(1.000000e-01);double(1.000000e-01);double(1.000000e-01);double(1.000000e-01);double(1.000000e-01);double(1.000000e-01);double(1.000000e-02);double(1.000000e-02);double(1.000000e-02);double(1.000000e-02);double(1.000000e-02);double(1.000000e-02);double(1.000000e-02);double(1.000000e-02);double(1.000000e-02);double(1.000000e-02);double(1.000000e-01);double(1.000000e-01);double(1.000000e-01);double(1.000000e-01);double(1.000000e-01);double(1.000000e-01);double(1.000000e-01);double(1.000000e-01);double(1.000000e-01);double(1.000000e-01);double(1.000000e-02);double(1.000000e-02);double(1.000000e-02);double(1.000000e-02);double(1.000000e-02);double(1.000000e-02);double(1.000000e-02);double(1.000000e-02);double(1.000000e-02);double(1.000000e-02)]')  Offsets=str2num('[double(0);double(0);double(0);double(0);double(0);double(0);double(0);double(0);double(0);double(0);double(0);double(0);double(0);double(0);double(0);double(0);double(0);double(0);double(0);double(0);double(0);double(0);double(0);double(0);double(0);double(0);double(0);double(0);double(0);double(0);double(0);double(0);double(0);double(0);double(0);double(0);double(0);double(0);double(0);double(0);double(1);double(1);double(1);double(1);double(1);double(1);double(1);double(1);double(1);double(1);double(0);double(0);double(0);double(0);double(0);double(0);double(0);double(0);double(0);double(0);double(0);double(0);double(0);double(0);double(0);double(0);double(0);double(0);double(0);double(0);double(0);double(0);double(0);double(0);double(0);double(0);double(0);double(0);double(0);double(0);double(0);double(0);double(0);double(0);double(0);double(0);double(0);double(0);double(0);double(0);double(0);double(-3.140000e+00);double(-3.140000e+00);double(-3.140000e+00);double(-3.140000e+00);double(-3.140000e+00);double(-3.140000e+00);double(-3.140000e+00);double(-3.140000e+00);double(-3.140000e+00);double(-3.140000e+00);double(0);double(0);double(0);double(0);double(0);double(0);double(0);double(0);double(0);double(0);double(0);double(0);double(0);double(0);double(0);double(0);double(0);double(0);double(0);double(0);double(0);double(0);double(0);double(0);double(0);double(0);double(0);double(0);double(0);double(0);double(-2.560000e+01);double(-2.560000e+01);double(-2.560000e+01);double(-2.560000e+01);double(-2.560000e+01);double(-2.560000e+01);double(-2.560000e+01);double(-2.560000e+01);double(-2.560000e+01);double(-2.560000e+01);double(0);double(0);double(0);double(0);double(0);double(0);double(0);double(0);double(0);double(0);double(-3.276800e+02);double(-3.276800e+02);double(-3.276800e+02);double(-3.276800e+02);double(-3.276800e+02);double(-3.276800e+02);double(-3.276800e+02);double(-3.276800e+02);double(-3.276800e+02);double(-3.276800e+02);double(0);double(0);double(0);double(0);double(0);double(0);double(0);double(0);double(0);double(0);double(-8.192000e+01);double(-8.192000e+01);double(-8.192000e+01);double(-8.192000e+01);double(-8.192000e+01);double(-8.192000e+01);double(-8.192000e+01);double(-8.192000e+01);double(-8.192000e+01);double(-8.192000e+01);double(0);double(0);double(0);double(0);double(0);double(0);double(0);double(0);double(0);double(0);double(-2.560000e+01);double(-2.560000e+01);double(-2.560000e+01);double(-2.560000e+01);double(-2.560000e+01);double(-2.560000e+01);double(-2.560000e+01);double(-2.560000e+01);double(-2.560000e+01);double(-2.560000e+01);double(0);double(0);double(0);double(0);double(0);double(0);double(0);double(0);double(0);double(0);double(-1.638400e+02);double(-1.638400e+02);double(-1.638400e+02);double(-1.638400e+02);double(-1.638400e+02);double(-1.638400e+02);double(-1.638400e+02);double(-1.638400e+02);double(-1.638400e+02);double(-1.638400e+02);double(0);double(0);double(0);double(0);double(0);double(0);double(0);double(0);double(0);double(0);double(-8.192000e+01);double(-8.192000e+01);double(-8.192000e+01);double(-8.192000e+01);double(-8.192000e+01);double(-8.192000e+01);double(-8.192000e+01);double(-8.192000e+01);double(-8.192000e+01);double(-8.192000e+01)]')  Minimums=str2num('[double(-Inf);double(-Inf);double(-Inf);double(-Inf);double(-Inf);double(-Inf);double(-Inf);double(-Inf);double(-Inf);double(-Inf);double(0);double(0);double(0);double(0);double(0);double(0);double(0);double(0);double(0);double(0);double(0);double(0);double(0);double(0);double(0);double(0);double(0);double(0);double(0);double(0);double(0);double(0);double(0);double(0);double(0);double(0);double(0);double(0);double(0);double(0);double(1);double(1);double(1);double(1);double(1);double(1);double(1);double(1);double(1);double(1);double(3.000000e-01);double(3.000000e-01);double(3.000000e-01);double(3.000000e-01);double(3.000000e-01);double(3.000000e-01);double(3.000000e-01);double(3.000000e-01);double(3.000000e-01);double(3.000000e-01);double(0);double(0);double(0);double(0);double(0);double(0);double(0);double(0);double(0);double(0);double(0);double(0);double(0);double(0);double(0);double(0);double(0);double(0);double(0);double(0);double(0);double(0);double(0);double(0);double(0);double(0);double(0);double(0);double(0);double(0);double(0);double(-3.140000e+00);double(-3.140000e+00);double(-3.140000e+00);double(-3.140000e+00);double(-3.140000e+00);double(-3.140000e+00);double(-3.140000e+00);double(-3.140000e+00);double(-3.140000e+00);double(-3.140000e+00);double(0);double(0);double(0);double(0);double(0);double(0);double(0);double(0);double(0);double(0);double(3.000000e-01);double(3.000000e-01);double(3.000000e-01);double(3.000000e-01);double(3.000000e-01);double(3.000000e-01);double(3.000000e-01);double(3.000000e-01);double(3.000000e-01);double(3.000000e-01);double(0);double(0);double(0);double(0);double(0);double(0);double(0);double(0);double(0);double(0);double(-2.560000e+01);double(-2.560000e+01);double(-2.560000e+01);double(-2.560000e+01);double(-2.560000e+01);double(-2.560000e+01);double(-2.560000e+01);double(-2.560000e+01);double(-2.560000e+01);double(-2.560000e+01);double(0);double(0);double(0);double(0);double(0);double(0);double(0);double(0);double(0);double(0);double(-3.276800e+02);double(-3.276800e+02);double(-3.276800e+02);double(-3.276800e+02);double(-3.276800e+02);double(-3.276800e+02);double(-3.276800e+02);double(-3.276800e+02);double(-3.276800e+02);double(-3.276800e+02);double(0);double(0);double(0);double(0);double(0);double(0);double(0);double(0);double(0);double(0);double(-8.192000e+01);double(-8.192000e+01);double(-8.192000e+01);double(-8.192000e+01);double(-8.192000e+01);double(-8.192000e+01);double(-8.192000e+01);double(-8.192000e+01);double(-8.192000e+01);double(-8.192000e+01);double(0);double(0);double(0);double(0);double(0);double(0);double(0);double(0);double(0);double(0);double(-2.560000e+01);double(-2.560000e+01);double(-2.560000e+01);double(-2.560000e+01);double(-2.560000e+01);double(-2.560000e+01);double(-2.560000e+01);double(-2.560000e+01);double(-2.560000e+01);double(-2.560000e+01);double(0);double(0);double(0);double(0);double(0);double(0);double(0);double(0);double(0);double(0);double(-1.638400e+02);double(-1.638400e+02);double(-1.638400e+02);double(-1.638400e+02);double(-1.638400e+02);double(-1.638400e+02);double(-1.638400e+02);double(-1.638400e+02);double(-1.638400e+02);double(-1.638400e+02);double(0);double(0);double(0);double(0);double(0);double(0);double(0);double(0);double(0);double(0);double(-8.192000e+01);double(-8.192000e+01);double(-8.192000e+01);double(-8.192000e+01);double(-8.192000e+01);double(-8.192000e+01);double(-8.192000e+01);double(-8.192000e+01);double(-8.192000e+01);double(-8.192000e+01)]')  Maximums=str2num('[double(Inf);double(Inf);double(Inf);double(Inf);double(Inf);double(Inf);double(Inf);double(Inf);double(Inf);double(Inf);double(7);double(7);double(7);double(7);double(7);double(7);double(7);double(7);double(7);double(7);double(1);double(1);double(1);double(1);double(1);double(1);double(1);double(1);double(1);double(1);double(5);double(5);double(5);double(5);double(5);double(5);double(5);double(5);double(5);double(5);double(1023);double(1023);double(1023);double(1023);double(1023);double(1023);double(1023);double(1023);double(1023);double(1023);double(5.140000e+01);double(5.140000e+01);double(5.140000e+01);double(5.140000e+01);double(5.140000e+01);double(5.140000e+01);double(5.140000e+01);double(5.140000e+01);double(5.140000e+01);double(5.140000e+01);double(15);double(15);double(15);double(15);double(15);double(15);double(15);double(15);double(15);double(15);double(255);double(1);double(1);double(1);double(1);double(1);double(1);double(1);double(1);double(1);double(1);double(1);double(1);double(1);double(1);double(1);double(1);double(1);double(1);double(1);double(1);double(3.140000e+00);double(3.140000e+00);double(3.140000e+00);double(3.140000e+00);double(3.140000e+00);double(3.140000e+00);double(3.140000e+00);double(3.140000e+00);double(3.140000e+00);double(3.140000e+00);double(9);double(9);double(9);double(9);double(9);double(9);double(9);double(9);double(9);double(9);double(3.300000e+00);double(3.300000e+00);double(3.300000e+00);double(3.300000e+00);double(3.300000e+00);double(3.300000e+00);double(3.300000e+00);double(3.300000e+00);double(3.300000e+00);double(3.300000e+00);double(5);double(5);double(5);double(5);double(5);double(5);double(5);double(5);double(5);double(5);double(2.550000e+01);double(2.550000e+01);double(2.550000e+01);double(2.550000e+01);double(2.550000e+01);double(2.550000e+01);double(2.550000e+01);double(2.550000e+01);double(2.550000e+01);double(2.550000e+01);double(25);double(25);double(25);double(25);double(25);double(25);double(25);double(25);double(25);double(25);double(3.276700e+02);double(3.276700e+02);double(3.276700e+02);double(3.276700e+02);double(3.276700e+02);double(3.276700e+02);double(3.276700e+02);double(3.276700e+02);double(3.276700e+02);double(3.276700e+02);double(15);double(15);double(15);double(15);double(15);double(15);double(15);double(15);double(15);double(15);double(8.191000e+01);double(8.191000e+01);double(8.191000e+01);double(8.191000e+01);double(8.191000e+01);double(8.191000e+01);double(8.191000e+01);double(8.191000e+01);double(8.191000e+01);double(8.191000e+01);double(5);double(5);double(5);double(5);double(5);double(5);double(5);double(5);double(5);double(5);double(2.550000e+01);double(2.550000e+01);double(2.550000e+01);double(2.550000e+01);double(2.550000e+01);double(2.550000e+01);double(2.550000e+01);double(2.550000e+01);double(2.550000e+01);double(2.550000e+01);double(25);double(25);double(25);double(25);double(25);double(25);double(25);double(25);double(25);double(25);double(1.638300e+02);double(1.638300e+02);double(1.638300e+02);double(1.638300e+02);double(1.638300e+02);double(1.638300e+02);double(1.638300e+02);double(1.638300e+02);double(1.638300e+02);double(1.638300e+02);double(15);double(15);double(15);double(15);double(15);double(15);double(15);double(15);double(15);double(15);double(8.191000e+01);double(8.191000e+01);double(8.191000e+01);double(8.191000e+01);double(8.191000e+01);double(8.191000e+01);double(8.191000e+01);double(8.191000e+01);double(8.191000e+01);double(8.191000e+01)]')  ApplyMinMax=off
      settings: SourceProductName=Simulink Real-Time  DataFormat=CANdb specified signals
  FLRdrObjInfo : Outport
  MValue : Outport  Port=2
  tag scope: ClassHighestProb_S2_001=global, ClassHighestProb_S2_002=global, ClassHighestProb_S2_003=global, ClassHighestProb_S2_004=global, ClassHighestProb_S2_005=global, ClassHighestProb_S2_006=global, ClassHighestProb_S2_007=global, ClassHighestProb_S2_008=global, ClassHighestProb_S2_009=global, ClassHighestProb_S2_010=global, ClassHighest_S2_001=global, ClassHighest_S2_002=global, ClassHighest_S2_003=global, ClassHighest_S2_004=global, ClassHighest_S2_005=global, ClassHighest_S2_006=global, ClassHighest_S2_007=global, ClassHighest_S2_008=global, ClassHighest_S2_009=global, ClassHighest_S2_010=global, ExistenceProb_S2_001=global, ExistenceProb_S2_002=global, ExistenceProb_S2_003=global, ExistenceProb_S2_004=global, ExistenceProb_S2_005=global, ExistenceProb_S2_006=global, ExistenceProb_S2_007=global, ExistenceProb_S2_008=global, ExistenceProb_S2_009=global, ExistenceProb_S2_010=global, Height_S2_001=global, Height_S2_002=global, Height_S2_003=global, Height_S2_004=global, Height_S2_005=global, Height_S2_006=global, Height_S2_007=global, Height_S2_008=global, Height_S2_009=global, Height_S2_010=global, Id_S2_001=global, Id_S2_002=global, Id_S2_003=global, Id_S2_004=global, Id_S2_005=global, Id_S2_006=global, Id_S2_007=global, Id_S2_008=global, Id_S2_009=global, Id_S2_010=global, Length_S2_001=global, Length_S2_002=global, Length_S2_003=global, Length_S2_004=global, Length_S2_005=global, Length_S2_006=global, Length_S2_007=global, Length_S2_008=global, Length_S2_009=global, Length_S2_010=global, MovingState_S2_001=global, MovingState_S2_002=global, MovingState_S2_003=global, MovingState_S2_004=global, MovingState_S2_005=global, MovingState_S2_006=global, MovingState_S2_007=global, MovingState_S2_008=global, MovingState_S2_009=global, MovingState_S2_010=global, ObjInit_S2_001=global, ObjInit_S2_002=global, ObjInit_S2_003=global, ObjInit_S2_004=global, ObjInit_S2_005=global, ObjInit_S2_006=global, ObjInit_S2_007=global, ObjInit_S2_008=global, ObjInit_S2_009=global, ObjInit_S2_010=global, ObjMeasured_S2_001=global, ObjMeasured_S2_002=global, ObjMeasured_S2_003=global, ObjMeasured_S2_004=global, ObjMeasured_S2_005=global, ObjMeasured_S2_006=global, ObjMeasured_S2_007=global, ObjMeasured_S2_008=global, ObjMeasured_S2_009=global, ObjMeasured_S2_010=global, Orientation_S2_001=global, Orientation_S2_002=global, Orientation_S2_003=global, Orientation_S2_004=global, Orientation_S2_005=global, Orientation_S2_006=global, Orientation_S2_007=global, Orientation_S2_008=global, Orientation_S2_009=global, Orientation_S2_010=global, ReferencePoint_S2_001=global, ReferencePoint_S2_002=global, ReferencePoint_S2_003=global, ReferencePoint_S2_004=global, ReferencePoint_S2_005=global, ReferencePoint_S2_006=global, ReferencePoint_S2_007=global, ReferencePoint_S2_008=global, ReferencePoint_S2_009=global, ReferencePoint_S2_010=global, Width_S2_001=global, Width_S2_002=global, Width_S2_003=global, Width_S2_004=global, Width_S2_005=global, Width_S2_006=global, Width_S2_007=global, Width_S2_008=global, Width_S2_009=global, Width_S2_010=global, XAccStd_S2_001=global, XAccStd_S2_002=global, XAccStd_S2_003=global, XAccStd_S2_004=global, XAccStd_S2_005=global, XAccStd_S2_006=global, XAccStd_S2_007=global, XAccStd_S2_008=global, XAccStd_S2_009=global, XAccStd_S2_010=global, XAcc_S2_001=global, XAcc_S2_002=global, XAcc_S2_003=global, XAcc_S2_004=global, XAcc_S2_005=global, XAcc_S2_006=global, XAcc_S2_007=global, XAcc_S2_008=global, XAcc_S2_009=global, XAcc_S2_010=global, XPosStd_S2_001=global, XPosStd_S2_002=global, XPosStd_S2_003=global, XPosStd_S2_004=global, XPosStd_S2_005=global, XPosStd_S2_006=global, XPosStd_S2_007=global, XPosStd_S2_008=global, XPosStd_S2_009=global, XPosStd_S2_010=global, XPos_S2_001=global, XPos_S2_002=global, XPos_S2_003=global, XPos_S2_004=global, XPos_S2_005=global, XPos_S2_006=global, XPos_S2_007=global, XPos_S2_008=global, XPos_S2_009=global, XPos_S2_010=global, XVelocityStd_S2_001=global, XVelocityStd_S2_002=global, XVelocityStd_S2_003=global, XVelocityStd_S2_004=global, XVelocityStd_S2_005=global, XVelocityStd_S2_006=global, XVelocityStd_S2_007=global, XVelocityStd_S2_008=global, XVelocityStd_S2_009=global, XVelocityStd_S2_010=global, XVelocity_S2_001=global, XVelocity_S2_002=global, XVelocity_S2_003=global, XVelocity_S2_004=global, XVelocity_S2_005=global, XVelocity_S2_006=global, XVelocity_S2_007=global, XVelocity_S2_008=global, XVelocity_S2_009=global, XVelocity_S2_010=global, YAccStd_S2_001=global, YAccStd_S2_002=global, YAccStd_S2_003=global, YAccStd_S2_004=global, YAccStd_S2_005=global, YAccStd_S2_006=global, YAccStd_S2_007=global, YAccStd_S2_008=global, YAccStd_S2_009=global, YAccStd_S2_010=global, YAcc_S2_001=global, YAcc_S2_002=global, YAcc_S2_003=global, YAcc_S2_004=global, YAcc_S2_005=global, YAcc_S2_006=global, YAcc_S2_007=global, YAcc_S2_008=global, YAcc_S2_009=global, YAcc_S2_010=global, YPosStd_S2_001=global, YPosStd_S2_002=global, YPosStd_S2_003=global, YPosStd_S2_004=global, YPosStd_S2_005=global, YPosStd_S2_006=global, YPosStd_S2_007=global, YPosStd_S2_008=global, YPosStd_S2_009=global, YPosStd_S2_010=global, YPos_S2_001=global, YPos_S2_002=global, YPos_S2_003=global, YPos_S2_004=global, YPos_S2_005=global, YPos_S2_006=global, YPos_S2_007=global, YPos_S2_008=global, YPos_S2_009=global, YPos_S2_010=global, YVelocityStd_S2_001=global, YVelocityStd_S2_002=global, YVelocityStd_S2_003=global, YVelocityStd_S2_004=global, YVelocityStd_S2_005=global, YVelocityStd_S2_006=global, YVelocityStd_S2_007=global, YVelocityStd_S2_008=global, YVelocityStd_S2_009=global, YVelocityStd_S2_010=global, YVelocity_S2_001=global, YVelocity_S2_002=global, YVelocity_S2_003=global, YVelocity_S2_004=global, YVelocity_S2_005=global, YVelocity_S2_006=global, YVelocity_S2_007=global, YVelocity_S2_008=global, YVelocity_S2_009=global, YVelocity_S2_010=global
  wires:
  msg/1 -> CAN FD Unpack3/1
  CAN FD Unpack3/41 -> [Id_S2_001]
  CAN FD Unpack3/42 -> [Id_S2_002]
  CAN FD Unpack3/43 -> [Id_S2_003]
  CAN FD Unpack3/44 -> [Id_S2_004]
  CAN FD Unpack3/45 -> [Id_S2_005]
  CAN FD Unpack3/46 -> [Id_S2_006]
  CAN FD Unpack3/47 -> [Id_S2_007]
  CAN FD Unpack3/48 -> [Id_S2_008]
  CAN FD Unpack3/49 -> [Id_S2_009]
  CAN FD Unpack3/50 -> [Id_S2_010]
  Bus Creator/1 -> FLRdrObjInfo/1  "FLRdrObjInfo"
  CAN FD Unpack3/71 -> [Multiplexor]
  CAN FD Unpack3/31 -> [Height_S2_001]
  CAN FD Unpack3/32 -> [Height_S2_002]
  CAN FD Unpack3/34 -> [Height_S2_004]
  CAN FD Unpack3/33 -> [Height_S2_003]
  CAN FD Unpack3/37 -> [Height_S2_007]
  CAN FD Unpack3/38 -> [Height_S2_008]
  CAN FD Unpack3/36 -> [Height_S2_006]
  CAN FD Unpack3/35 -> [Height_S2_005]
  CAN FD Unpack3/40 -> [Height_S2_010]
  CAN FD Unpack3/39 -> [Height_S2_009]
  CAN FD Unpack3/30 -> [ExistenceProb_S2_010]
  CAN FD Unpack3/20 -> [ClassHighest_S2_010]
  CAN FD Unpack3/21 -> [ExistenceProb_S2_001]
  CAN FD Unpack3/22 -> [ExistenceProb_S2_002]
  CAN FD Unpack3/23 -> [ExistenceProb_S2_003]
  CAN FD Unpack3/24 -> [ExistenceProb_S2_004]
  CAN FD Unpack3/28 -> [ExistenceProb_S2_008]
  CAN FD Unpack3/27 -> [ExistenceProb_S2_007]
  CAN FD Unpack3/26 -> [ExistenceProb_S2_006]
  CAN FD Unpack3/25 -> [ExistenceProb_S2_005]
  CAN FD Unpack3/29 -> [ExistenceProb_S2_009]
  CAN FD Unpack3/11 -> [ClassHighest_S2_001]
  CAN FD Unpack3/12 -> [ClassHighest_S2_002]
  CAN FD Unpack3/14 -> [ClassHighest_S2_004]
  CAN FD Unpack3/13 -> [ClassHighest_S2_003]
  CAN FD Unpack3/17 -> [ClassHighest_S2_007]
  CAN FD Unpack3/18 -> [ClassHighest_S2_008]
  CAN FD Unpack3/16 -> [ClassHighest_S2_006]
  CAN FD Unpack3/15 -> [ClassHighest_S2_005]
  CAN FD Unpack3/19 -> [ClassHighest_S2_009]
  CAN FD Unpack3/1 -> [ClassHighestProb_S2_001]
  CAN FD Unpack3/2 -> [ClassHighestProb_S2_002]
  CAN FD Unpack3/4 -> [ClassHighestProb_S2_004]
  CAN FD Unpack3/3 -> [ClassHighestProb_S2_003]
  CAN FD Unpack3/7 -> [ClassHighestProb_S2_007]
  CAN FD Unpack3/8 -> [ClassHighestProb_S2_008]
  CAN FD Unpack3/6 -> [ClassHighestProb_S2_006]
  CAN FD Unpack3/5 -> [ClassHighestProb_S2_005]
  CAN FD Unpack3/10 -> [ClassHighestProb_S2_010]
  CAN FD Unpack3/9 -> [ClassHighestProb_S2_009]
  CAN FD Unpack3/51 -> [Length_S2_001]
  CAN FD Unpack3/52 -> [Length_S2_002]
  CAN FD Unpack3/54 -> [Length_S2_004]
  CAN FD Unpack3/53 -> [Length_S2_003]
  CAN FD Unpack3/57 -> [Length_S2_007]
  CAN FD Unpack3/58 -> [Length_S2_008]
  CAN FD Unpack3/56 -> [Length_S2_006]
  CAN FD Unpack3/55 -> [Length_S2_005]
  CAN FD Unpack3/61 -> [MovingState_S2_001]
  CAN FD Unpack3/60 -> [Length_S2_010]
  CAN FD Unpack3/59 -> [Length_S2_009]
  CAN FD Unpack3/62 -> [MovingState_S2_002]
  CAN FD Unpack3/64 -> [MovingState_S2_004]
  CAN FD Unpack3/63 -> [MovingState_S2_003]
  CAN FD Unpack3/67 -> [MovingState_S2_007]
  CAN FD Unpack3/68 -> [MovingState_S2_008]
  CAN FD Unpack3/66 -> [MovingState_S2_006]
  CAN FD Unpack3/65 -> [MovingState_S2_005]
  CAN FD Unpack3/70 -> [MovingState_S2_010]
  CAN FD Unpack3/69 -> [MovingState_S2_009]
  CAN FD Unpack3/72 -> [ObjInit_S2_001]
  CAN FD Unpack3/73 -> [ObjInit_S2_002]
  CAN FD Unpack3/75 -> [ObjInit_S2_004]
  CAN FD Unpack3/74 -> [ObjInit_S2_003]
  CAN FD Unpack3/78 -> [ObjInit_S2_007]
  CAN FD Unpack3/79 -> [ObjInit_S2_008]
  CAN FD Unpack3/77 -> [ObjInit_S2_006]
  CAN FD Unpack3/76 -> [ObjInit_S2_005]
  CAN FD Unpack3/81 -> [ObjInit_S2_010]
  CAN FD Unpack3/80 -> [ObjInit_S2_009]
  CAN FD Unpack3/82 -> [ObjMeasured_S2_001]
  CAN FD Unpack3/83 -> [ObjMeasured_S2_002]
  CAN FD Unpack3/85 -> [ObjMeasured_S2_004]
  CAN FD Unpack3/84 -> [ObjMeasured_S2_003]
  CAN FD Unpack3/88 -> [ObjMeasured_S2_007]
  CAN FD Unpack3/89 -> [ObjMeasured_S2_008]
  CAN FD Unpack3/87 -> [ObjMeasured_S2_006]
  CAN FD Unpack3/86 -> [ObjMeasured_S2_005]
  CAN FD Unpack3/90 -> [ObjMeasured_S2_009]
  CAN FD Unpack3/92 -> [Orientation_S2_001]
  CAN FD Unpack3/91 -> [ObjMeasured_S2_010]
  CAN FD Unpack3/93 -> [Orientation_S2_002]
  CAN FD Unpack3/95 -> [Orientation_S2_004]
  CAN FD Unpack3/94 -> [Orientation_S2_003]
  CAN FD Unpack3/98 -> [Orientation_S2_007]
  CAN FD Unpack3/99 -> [Orientation_S2_008]
  CAN FD Unpack3/97 -> [Orientation_S2_006]
  CAN FD Unpack3/96 -> [Orientation_S2_005]
  CAN FD Unpack3/100 -> [Orientation_S2_009]
  CAN FD Unpack3/102 -> [ReferencePoint_S2_001]
  CAN FD Unpack3/101 -> [Orientation_S2_010]
  CAN FD Unpack3/103 -> [ReferencePoint_S2_002]
  CAN FD Unpack3/105 -> [ReferencePoint_S2_004]
  CAN FD Unpack3/104 -> [ReferencePoint_S2_003]
  CAN FD Unpack3/108 -> [ReferencePoint_S2_007]
  CAN FD Unpack3/109 -> [ReferencePoint_S2_008]
  CAN FD Unpack3/107 -> [ReferencePoint_S2_006]
  CAN FD Unpack3/106 -> [ReferencePoint_S2_005]
  CAN FD Unpack3/110 -> [ReferencePoint_S2_009]
  CAN FD Unpack3/112 -> [Width_S2_001]
  CAN FD Unpack3/111 -> [ReferencePoint_S2_010]
  CAN FD Unpack3/113 -> [Width_S2_002]
  CAN FD Unpack3/115 -> [Width_S2_004]
  CAN FD Unpack3/114 -> [Width_S2_003]
  CAN FD Unpack3/118 -> [Width_S2_007]
  CAN FD Unpack3/119 -> [Width_S2_008]
  CAN FD Unpack3/117 -> [Width_S2_006]
  CAN FD Unpack3/116 -> [Width_S2_005]
  CAN FD Unpack3/120 -> [Width_S2_009]
  CAN FD Unpack3/122 -> [XAccStd_S2_001]
  CAN FD Unpack3/121 -> [Width_S2_010]
  CAN FD Unpack3/123 -> [XAccStd_S2_002]
  CAN FD Unpack3/125 -> [XAccStd_S2_004]
  CAN FD Unpack3/124 -> [XAccStd_S2_003]
  CAN FD Unpack3/128 -> [XAccStd_S2_007]
  CAN FD Unpack3/129 -> [XAccStd_S2_008]
  CAN FD Unpack3/127 -> [XAccStd_S2_006]
  CAN FD Unpack3/126 -> [XAccStd_S2_005]
  CAN FD Unpack3/130 -> [XAccStd_S2_009]
  CAN FD Unpack3/131 -> [XAccStd_S2_010]
  CAN FD Unpack3/141 -> [XAcc_S2_010]
  CAN FD Unpack3/140 -> [XAcc_S2_009]
  CAN FD Unpack3/136 -> [XAcc_S2_005]
  CAN FD Unpack3/137 -> [XAcc_S2_006]
  CAN FD Unpack3/139 -> [XAcc_S2_008]
  CAN FD Unpack3/138 -> [XAcc_S2_007]
  CAN FD Unpack3/134 -> [XAcc_S2_003]
  CAN FD Unpack3/135 -> [XAcc_S2_004]
  CAN FD Unpack3/133 -> [XAcc_S2_002]
  CAN FD Unpack3/132 -> [XAcc_S2_001]
  CAN FD Unpack3/142 -> [XPosStd_S2_001]
  CAN FD Unpack3/143 -> [XPosStd_S2_002]
  CAN FD Unpack3/145 -> [XPosStd_S2_004]
  CAN FD Unpack3/144 -> [XPosStd_S2_003]
  CAN FD Unpack3/148 -> [XPosStd_S2_007]
  CAN FD Unpack3/149 -> [XPosStd_S2_008]
  CAN FD Unpack3/147 -> [XPosStd_S2_006]
  CAN FD Unpack3/146 -> [XPosStd_S2_005]
  CAN FD Unpack3/151 -> [XPosStd_S2_010]
  CAN FD Unpack3/150 -> [XPosStd_S2_009]
  CAN FD Unpack3/160 -> [XPos_S2_009]
  CAN FD Unpack3/161 -> [XPos_S2_010]
  CAN FD Unpack3/156 -> [XPos_S2_005]
  CAN FD Unpack3/157 -> [XPos_S2_006]
  CAN FD Unpack3/159 -> [XPos_S2_008]
  CAN FD Unpack3/158 -> [XPos_S2_007]
  CAN FD Unpack3/154 -> [XPos_S2_003]
  CAN FD Unpack3/155 -> [XPos_S2_004]
  CAN FD Unpack3/153 -> [XPos_S2_002]
  CAN FD Unpack3/152 -> [XPos_S2_001]
  CAN FD Unpack3/162 -> [XVelocityStd_S2_001]
  CAN FD Unpack3/163 -> [XVelocityStd_S2_002]
  CAN FD Unpack3/165 -> [XVelocityStd_S2_004]
  CAN FD Unpack3/164 -> [XVelocityStd_S2_003]
  CAN FD Unpack3/168 -> [XVelocityStd_S2_007]
  CAN FD Unpack3/169 -> [XVelocityStd_S2_008]
  CAN FD Unpack3/167 -> [XVelocityStd_S2_006]
  CAN FD Unpack3/166 -> [XVelocityStd_S2_005]
  CAN FD Unpack3/171 -> [XVelocityStd_S2_010]
  CAN FD Unpack3/170 -> [XVelocityStd_S2_009]
  CAN FD Unpack3/180 -> [XVelocity_S2_009]
  CAN FD Unpack3/181 -> [XVelocity_S2_010]
  CAN FD Unpack3/176 -> [XVelocity_S2_005]
  CAN FD Unpack3/177 -> [XVelocity_S2_006]
  CAN FD Unpack3/179 -> [XVelocity_S2_008]
  CAN FD Unpack3/178 -> [XVelocity_S2_007]
  CAN FD Unpack3/174 -> [XVelocity_S2_003]
  CAN FD Unpack3/175 -> [XVelocity_S2_004]
  CAN FD Unpack3/173 -> [XVelocity_S2_002]
  CAN FD Unpack3/172 -> [XVelocity_S2_001]
  CAN FD Unpack3/232 -> [YVelocity_S2_001]
  CAN FD Unpack3/233 -> [YVelocity_S2_002]
  CAN FD Unpack3/235 -> [YVelocity_S2_004]
  CAN FD Unpack3/234 -> [YVelocity_S2_003]
  CAN FD Unpack3/238 -> [YVelocity_S2_007]
  CAN FD Unpack3/239 -> [YVelocity_S2_008]
  CAN FD Unpack3/237 -> [YVelocity_S2_006]
  CAN FD Unpack3/236 -> [YVelocity_S2_005]
  CAN FD Unpack3/241 -> [YVelocity_S2_010]
  CAN FD Unpack3/240 -> [YVelocity_S2_009]
  CAN FD Unpack3/230 -> [YVelocityStd_S2_009]
  CAN FD Unpack3/231 -> [YVelocityStd_S2_010]
  CAN FD Unpack3/226 -> [YVelocityStd_S2_005]
  CAN FD Unpack3/227 -> [YVelocityStd_S2_006]
  CAN FD Unpack3/229 -> [YVelocityStd_S2_008]
  CAN FD Unpack3/228 -> [YVelocityStd_S2_007]
  CAN FD Unpack3/224 -> [YVelocityStd_S2_003]
  CAN FD Unpack3/225 -> [YVelocityStd_S2_004]
  CAN FD Unpack3/223 -> [YVelocityStd_S2_002]
  CAN FD Unpack3/222 -> [YVelocityStd_S2_001]
  CAN FD Unpack3/212 -> [YPos_S2_001]
  CAN FD Unpack3/213 -> [YPos_S2_002]
  CAN FD Unpack3/215 -> [YPos_S2_004]
  CAN FD Unpack3/214 -> [YPos_S2_003]
  CAN FD Unpack3/218 -> [YPos_S2_007]
  CAN FD Unpack3/219 -> [YPos_S2_008]
  CAN FD Unpack3/217 -> [YPos_S2_006]
  CAN FD Unpack3/216 -> [YPos_S2_005]
  CAN FD Unpack3/221 -> [YPos_S2_010]
  CAN FD Unpack3/220 -> [YPos_S2_009]
  CAN FD Unpack3/210 -> [YPosStd_S2_009]
  CAN FD Unpack3/211 -> [YPosStd_S2_010]
  CAN FD Unpack3/206 -> [YPosStd_S2_005]
  CAN FD Unpack3/207 -> [YPosStd_S2_006]
  CAN FD Unpack3/209 -> [YPosStd_S2_008]
  CAN FD Unpack3/208 -> [YPosStd_S2_007]
  CAN FD Unpack3/204 -> [YPosStd_S2_003]
  CAN FD Unpack3/205 -> [YPosStd_S2_004]
  CAN FD Unpack3/203 -> [YPosStd_S2_002]
  CAN FD Unpack3/202 -> [YPosStd_S2_001]
  CAN FD Unpack3/192 -> [YAcc_S2_001]
  CAN FD Unpack3/193 -> [YAcc_S2_002]
  CAN FD Unpack3/195 -> [YAcc_S2_004]
  CAN FD Unpack3/194 -> [YAcc_S2_003]
  CAN FD Unpack3/198 -> [YAcc_S2_007]
  CAN FD Unpack3/199 -> [YAcc_S2_008]
  CAN FD Unpack3/197 -> [YAcc_S2_006]
  CAN FD Unpack3/196 -> [YAcc_S2_005]
  CAN FD Unpack3/200 -> [YAcc_S2_009]
  CAN FD Unpack3/201 -> [YAcc_S2_010]
  CAN FD Unpack3/191 -> [YAccStd_S2_010]
  CAN FD Unpack3/190 -> [YAccStd_S2_009]
  CAN FD Unpack3/186 -> [YAccStd_S2_005]
  CAN FD Unpack3/187 -> [YAccStd_S2_006]
  CAN FD Unpack3/189 -> [YAccStd_S2_008]
  CAN FD Unpack3/188 -> [YAccStd_S2_007]
  CAN FD Unpack3/184 -> [YAccStd_S2_003]
  CAN FD Unpack3/185 -> [YAccStd_S2_004]
  CAN FD Unpack3/183 -> [YAccStd_S2_002]
  CAN FD Unpack3/182 -> [YAccStd_S2_001]
  [Id_S2_001] -> Bus Creator1/1
  [ObjInit_S2_001] -> Bus Creator1/2
  [ObjMeasured_S2_001] -> Bus Creator1/3
  [XPos_S2_001] -> Bus Creator1/4
  [YPos_S2_001] -> Bus Creator1/5
  [XVelocity_S2_001] -> Bus Creator1/6
  [YVelocity_S2_001] -> Bus Creator1/7
  [XAcc_S2_001] -> Bus Creator1/8
  [YAcc_S2_001] -> Bus Creator1/9
  [Width_S2_001] -> Bus Creator1/10
  [Length_S2_001] -> Bus Creator1/11
  [Orientation_S2_001] -> Bus Creator1/12
  [ExistenceProb_S2_001] -> Bus Creator1/13
  [MovingState_S2_001] -> Bus Creator1/14
  [ClassHighest_S2_001] -> Bus Creator1/15
  [ClassHighestProb_S2_001] -> Bus Creator1/16
  [ReferencePoint_S2_001] -> Bus Creator1/17
  [Height_S2_001] -> Bus Creator1/18
  [XAccStd_S2_001] -> Bus Creator1/19
  [XPosStd_S2_001] -> Bus Creator1/20
  [XVelocityStd_S2_001] -> Bus Creator1/21
  [YAccStd_S2_001] -> Bus Creator1/22
  [YPosStd_S2_001] -> Bus Creator1/23
  [YVelocityStd_S2_001] -> Bus Creator1/24
  Bus Creator1/1 -> [Obj1Info]  "Obj1Info"
  Bus Creator2/1 -> [Obj2Info]  "Obj2Info"
  [YVelocityStd_S2_002] -> Bus Creator2/24
  [YPosStd_S2_002] -> Bus Creator2/23
  [YAccStd_S2_002] -> Bus Creator2/22
  [XVelocityStd_S2_002] -> Bus Creator2/21
  [XPosStd_S2_002] -> Bus Creator2/20
  [XAccStd_S2_002] -> Bus Creator2/19
  [Height_S2_002] -> Bus Creator2/18
  [ReferencePoint_S2_002] -> Bus Creator2/17
  [ClassHighestProb_S2_002] -> Bus Creator2/16
  [ClassHighest_S2_002] -> Bus Creator2/15
  [MovingState_S2_002] -> Bus Creator2/14
  [ExistenceProb_S2_002] -> Bus Creator2/13
  [Orientation_S2_002] -> Bus Creator2/12
  [Length_S2_002] -> Bus Creator2/11
  [Width_S2_002] -> Bus Creator2/10
  [YAcc_S2_002] -> Bus Creator2/9
  [XAcc_S2_002] -> Bus Creator2/8
  [YVelocity_S2_002] -> Bus Creator2/7
  [XVelocity_S2_002] -> Bus Creator2/6
  [YPos_S2_002] -> Bus Creator2/5
  [XPos_S2_002] -> Bus Creator2/4
  [ObjMeasured_S2_002] -> Bus Creator2/3
  [ObjInit_S2_002] -> Bus Creator2/2
  [Id_S2_002] -> Bus Creator2/1
  [Id_S2_003] -> Bus Creator3/1
  [ObjInit_S2_003] -> Bus Creator3/2
  [ObjMeasured_S2_003] -> Bus Creator3/3
  [XPos_S2_003] -> Bus Creator3/4
  [YPos_S2_003] -> Bus Creator3/5
  [XVelocity_S2_003] -> Bus Creator3/6
  [YVelocity_S2_003] -> Bus Creator3/7
  [XAcc_S2_003] -> Bus Creator3/8
  [YAcc_S2_003] -> Bus Creator3/9
  [Width_S2_003] -> Bus Creator3/10
  [Length_S2_003] -> Bus Creator3/11
  [Orientation_S2_003] -> Bus Creator3/12
  [ExistenceProb_S2_003] -> Bus Creator3/13
  [MovingState_S2_003] -> Bus Creator3/14
  [ClassHighest_S2_003] -> Bus Creator3/15
  [ClassHighestProb_S2_003] -> Bus Creator3/16
  [ReferencePoint_S2_003] -> Bus Creator3/17
  [Height_S2_003] -> Bus Creator3/18
  [XAccStd_S2_003] -> Bus Creator3/19
  [XPosStd_S2_003] -> Bus Creator3/20
  [XVelocityStd_S2_003] -> Bus Creator3/21
  [YAccStd_S2_003] -> Bus Creator3/22
  [YPosStd_S2_003] -> Bus Creator3/23
  [YVelocityStd_S2_003] -> Bus Creator3/24
  Bus Creator3/1 -> [Obj3Info]  "Obj3Info"
  Bus Creator4/1 -> [Obj4Info]  "Obj4Info"
  [YVelocityStd_S2_004] -> Bus Creator4/24
  [YPosStd_S2_004] -> Bus Creator4/23
  [YAccStd_S2_004] -> Bus Creator4/22
  [XVelocityStd_S2_004] -> Bus Creator4/21
  [XPosStd_S2_004] -> Bus Creator4/20
  [XAccStd_S2_004] -> Bus Creator4/19
  [Height_S2_004] -> Bus Creator4/18
  [ReferencePoint_S2_004] -> Bus Creator4/17
  [ClassHighestProb_S2_004] -> Bus Creator4/16
  [ClassHighest_S2_004] -> Bus Creator4/15
  [MovingState_S2_004] -> Bus Creator4/14
  [ExistenceProb_S2_004] -> Bus Creator4/13
  [Orientation_S2_004] -> Bus Creator4/12
  [Length_S2_004] -> Bus Creator4/11
  [Width_S2_004] -> Bus Creator4/10
  [YAcc_S2_004] -> Bus Creator4/9
  [XAcc_S2_004] -> Bus Creator4/8
  [YVelocity_S2_004] -> Bus Creator4/7
  [XVelocity_S2_004] -> Bus Creator4/6
  [YPos_S2_004] -> Bus Creator4/5
  [XPos_S2_004] -> Bus Creator4/4
  [ObjMeasured_S2_004] -> Bus Creator4/3
  [ObjInit_S2_004] -> Bus Creator4/2
  [Id_S2_004] -> Bus Creator4/1
  [Id_S2_005] -> Bus Creator5/1
  [ObjInit_S2_005] -> Bus Creator5/2
  [ObjMeasured_S2_005] -> Bus Creator5/3
  [XPos_S2_005] -> Bus Creator5/4
  [YPos_S2_005] -> Bus Creator5/5
  [XVelocity_S2_005] -> Bus Creator5/6
  [YVelocity_S2_005] -> Bus Creator5/7
  [XAcc_S2_005] -> Bus Creator5/8
  [YAcc_S2_005] -> Bus Creator5/9
  [Width_S2_005] -> Bus Creator5/10
  [Length_S2_005] -> Bus Creator5/11
  [Orientation_S2_005] -> Bus Creator5/12
  [ExistenceProb_S2_005] -> Bus Creator5/13
  [MovingState_S2_005] -> Bus Creator5/14
  [ClassHighest_S2_005] -> Bus Creator5/15
  [ClassHighestProb_S2_005] -> Bus Creator5/16
  [ReferencePoint_S2_005] -> Bus Creator5/17
  [Height_S2_005] -> Bus Creator5/18
  [XAccStd_S2_005] -> Bus Creator5/19
  [XPosStd_S2_005] -> Bus Creator5/20
  [XVelocityStd_S2_005] -> Bus Creator5/21
  [YAccStd_S2_005] -> Bus Creator5/22
  [YPosStd_S2_005] -> Bus Creator5/23
  [YVelocityStd_S2_005] -> Bus Creator5/24
  Bus Creator5/1 -> [Obj5Info]  "Obj5Info"
  Bus Creator10/1 -> [Obj10Info]  "Obj10Info"
  [YVelocityStd_S2_010] -> Bus Creator10/24
  [YPosStd_S2_010] -> Bus Creator10/23
  [YAccStd_S2_010] -> Bus Creator10/22
  [XVelocityStd_S2_010] -> Bus Creator10/21
  [XPosStd_S2_010] -> Bus Creator10/20
  [XAccStd_S2_010] -> Bus Creator10/19
  [Height_S2_010] -> Bus Creator10/18
  [ReferencePoint_S2_010] -> Bus Creator10/17
  [ClassHighestProb_S2_010] -> Bus Creator10/16
  [ClassHighest_S2_010] -> Bus Creator10/15
  [MovingState_S2_010] -> Bus Creator10/14
  [ExistenceProb_S2_010] -> Bus Creator10/13
  [Orientation_S2_010] -> Bus Creator10/12
  [Length_S2_010] -> Bus Creator10/11
  [Width_S2_010] -> Bus Creator10/10
  [YAcc_S2_010] -> Bus Creator10/9
  [XAcc_S2_010] -> Bus Creator10/8
  [YVelocity_S2_010] -> Bus Creator10/7
  [XVelocity_S2_010] -> Bus Creator10/6
  [YPos_S2_010] -> Bus Creator10/5
  [XPos_S2_010] -> Bus Creator10/4
  [ObjMeasured_S2_010] -> Bus Creator10/3
  [ObjInit_S2_010] -> Bus Creator10/2
  [Id_S2_010] -> Bus Creator10/1
  [Id_S2_009] -> Bus Creator9/1
  [ObjInit_S2_009] -> Bus Creator9/2
  [ObjMeasured_S2_009] -> Bus Creator9/3
  [XPos_S2_009] -> Bus Creator9/4
  [YPos_S2_009] -> Bus Creator9/5
  [XVelocity_S2_009] -> Bus Creator9/6
  [YVelocity_S2_009] -> Bus Creator9/7
  [XAcc_S2_009] -> Bus Creator9/8
  [YAcc_S2_009] -> Bus Creator9/9
  [Width_S2_009] -> Bus Creator9/10
  [Length_S2_009] -> Bus Creator9/11
  [Orientation_S2_009] -> Bus Creator9/12
  [ExistenceProb_S2_009] -> Bus Creator9/13
  [MovingState_S2_009] -> Bus Creator9/14
  [ClassHighest_S2_009] -> Bus Creator9/15
  [ClassHighestProb_S2_009] -> Bus Creator9/16
  [ReferencePoint_S2_009] -> Bus Creator9/17
  [Height_S2_009] -> Bus Creator9/18
  [XAccStd_S2_009] -> Bus Creator9/19
  [XPosStd_S2_009] -> Bus Creator9/20
  [XVelocityStd_S2_009] -> Bus Creator9/21
  [YAccStd_S2_009] -> Bus Creator9/22
  [YPosStd_S2_009] -> Bus Creator9/23
  [YVelocityStd_S2_009] -> Bus Creator9/24
  Bus Creator9/1 -> [Obj9Info]  "Obj9Info"
  Bus Creator8/1 -> [Obj8Info]  "Obj8Info"
  [YVelocityStd_S2_008] -> Bus Creator8/24
  [YPosStd_S2_008] -> Bus Creator8/23
  [YAccStd_S2_008] -> Bus Creator8/22
  [XVelocityStd_S2_008] -> Bus Creator8/21
  [XPosStd_S2_008] -> Bus Creator8/20
  [XAccStd_S2_008] -> Bus Creator8/19
  [Height_S2_008] -> Bus Creator8/18
  [ReferencePoint_S2_008] -> Bus Creator8/17
  [ClassHighestProb_S2_008] -> Bus Creator8/16
  [ClassHighest_S2_008] -> Bus Creator8/15
  [MovingState_S2_008] -> Bus Creator8/14
  [ExistenceProb_S2_008] -> Bus Creator8/13
  [Orientation_S2_008] -> Bus Creator8/12
  [Length_S2_008] -> Bus Creator8/11
  [Width_S2_008] -> Bus Creator8/10
  [YAcc_S2_008] -> Bus Creator8/9
  [XAcc_S2_008] -> Bus Creator8/8
  [YVelocity_S2_008] -> Bus Creator8/7
  [XVelocity_S2_008] -> Bus Creator8/6
  [YPos_S2_008] -> Bus Creator8/5
  [XPos_S2_008] -> Bus Creator8/4
  [ObjMeasured_S2_008] -> Bus Creator8/3
  [ObjInit_S2_008] -> Bus Creator8/2
  [Id_S2_008] -> Bus Creator8/1
  [Id_S2_007] -> Bus Creator7/1
  [ObjInit_S2_007] -> Bus Creator7/2
  [ObjMeasured_S2_007] -> Bus Creator7/3
  [XPos_S2_007] -> Bus Creator7/4
  [YPos_S2_007] -> Bus Creator7/5
  [XVelocity_S2_007] -> Bus Creator7/6
  [YVelocity_S2_007] -> Bus Creator7/7
  [XAcc_S2_007] -> Bus Creator7/8
  [YAcc_S2_007] -> Bus Creator7/9
  [Width_S2_007] -> Bus Creator7/10
  [Length_S2_007] -> Bus Creator7/11
  [Orientation_S2_007] -> Bus Creator7/12
  [ExistenceProb_S2_007] -> Bus Creator7/13
  [MovingState_S2_007] -> Bus Creator7/14
  [ClassHighest_S2_007] -> Bus Creator7/15
  [ClassHighestProb_S2_007] -> Bus Creator7/16
  [ReferencePoint_S2_007] -> Bus Creator7/17
  [Height_S2_007] -> Bus Creator7/18
  [XAccStd_S2_007] -> Bus Creator7/19
  [XPosStd_S2_007] -> Bus Creator7/20
  [XVelocityStd_S2_007] -> Bus Creator7/21
  [YAccStd_S2_007] -> Bus Creator7/22
  [YPosStd_S2_007] -> Bus Creator7/23
  [YVelocityStd_S2_007] -> Bus Creator7/24
  Bus Creator7/1 -> [Obj7Info]  "Obj7Info"
  Bus Creator6/1 -> [Obj6Info]  "Obj6Info"
  [YVelocityStd_S2_006] -> Bus Creator6/24
  [YPosStd_S2_006] -> Bus Creator6/23
  [YAccStd_S2_006] -> Bus Creator6/22
  [XVelocityStd_S2_006] -> Bus Creator6/21
  [XPosStd_S2_006] -> Bus Creator6/20
  [XAccStd_S2_006] -> Bus Creator6/19
  [Height_S2_006] -> Bus Creator6/18
  [ReferencePoint_S2_006] -> Bus Creator6/17
  [ClassHighestProb_S2_006] -> Bus Creator6/16
  [ClassHighest_S2_006] -> Bus Creator6/15
  [MovingState_S2_006] -> Bus Creator6/14
  [ExistenceProb_S2_006] -> Bus Creator6/13
  [Orientation_S2_006] -> Bus Creator6/12
  [Length_S2_006] -> Bus Creator6/11
  [Width_S2_006] -> Bus Creator6/10
  [YAcc_S2_006] -> Bus Creator6/9
  [XAcc_S2_006] -> Bus Creator6/8
  [YVelocity_S2_006] -> Bus Creator6/7
  [XVelocity_S2_006] -> Bus Creator6/6
  [YPos_S2_006] -> Bus Creator6/5
  [XPos_S2_006] -> Bus Creator6/4
  [ObjMeasured_S2_006] -> Bus Creator6/3
  [ObjInit_S2_006] -> Bus Creator6/2
  [Id_S2_006] -> Bus Creator6/1
  [Obj1Info] -> Bus Creator/1
  [Obj2Info] -> Bus Creator/2
  [Obj3Info] -> Bus Creator/3
  [Obj4Info] -> Bus Creator/4
  [Obj6Info] -> Bus Creator/6
  [Obj5Info] -> Bus Creator/5
  [Obj7Info] -> Bus Creator/7
  [Obj8Info] -> Bus Creator/8
  [Obj9Info] -> Bus Creator/9
  [Obj10Info] -> Bus Creator/10
  [Multiplexor] -> MValue/1
